simulink model "test_convert"  (Simulink 6.2)
settings: Solver=ode45  StartTime=0.0  StopTime=10.0  RelTol=1e-3
libraries: xbsIndex_r3 x9
settings Model: LastModifiedBy=mdexter
settings DebuggingCC: SolverPrmCheckMsg=warning

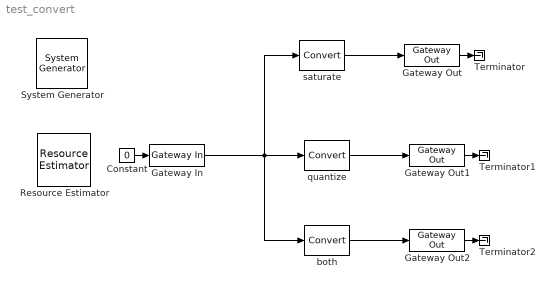
== system test_convert ==
  " System Generator" : xbsIndex_r3/ System Generator  Tag=genX  xilinxfamily=Virtex2  part=xc2v1000  speed=-4  package=bg575  synthesis_tool=XST  directory=./test_convert.netlist  testbench=off  simulink_period=1  sysclk_period=100  incr_netlist=off  trim_vbits=Everywhere in SubSystem  dbl_ovrd=According to Block Masks  core_generation=According to Block Masks  run_coregen=off  deprecated_control=off  eval_field=0
      settings: AttributesFormatString=System\nGenerator
  Constant : Constant  Value=0
  Gateway In : xbsIndex_r3/Gateway In  arith_type="Signed  (2's comp)"  n_bits=18  bin_pt=9  quantization=Truncate  overflow=Wrap  period=1  timing_constraint=None  locs_specified=off  LOCs={}  needs_fixed_name=off  dbl_ovrd=off  show_param=off
      settings: xl_area=[0 0 0 0 18 0 0]
  Gateway Out : xbsIndex_r3/Gateway Out  output_type=Double  nbits=8  bin_pt=6  arith_type=Boolean  quantization=Truncate  overflow=Wrap  hdl_port=on  timing_constraint=None  locs_specified=off  LOCs={}  needs_fixed_name=off  show_param=off
      settings: xl_area=[0 0 0 0 10 0 0]
  Gateway Out1 : xbsIndex_r3/Gateway Out  output_type=Double  nbits=8  bin_pt=6  arith_type=Boolean  quantization=Truncate  overflow=Wrap  hdl_port=on  timing_constraint=None  locs_specified=off  LOCs={}  needs_fixed_name=off  show_param=off
      settings: xl_area=[0 0 0 0 9 0 0]
  Gateway Out2 : xbsIndex_r3/Gateway Out  output_type=Double  nbits=8  bin_pt=6  arith_type=Boolean  quantization=Truncate  overflow=Wrap  hdl_port=on  timing_constraint=None  locs_specified=off  LOCs={}  needs_fixed_name=off  show_param=off
      settings: xl_area=[0 0 0 0 4 0 0]
  Resource Estimator : xbsIndex_r3/Resource Estimator  Tag=resEstTag  xl_estimator_area=[39 23 0 71 41 0 0]  xl_use_estimator_area=off  simulink_period=1  mrp_directory=./bitsel_core
      settings: AttributesFormatString=Resource\nEstimator
  Terminator : Terminator
  Terminator1 : Terminator
  Terminator2 : Terminator
  both : xbsIndex_r3/Convert  arith_type="Signed  (2's comp)"  n_bits=4  bin_pt=0  quantization="Round  (unbiased: Even Values)"  overflow=Saturate  latency=3  explicit_period=off  period=1  dbl_ovrd=off  show_param=on  inserted_by_tool=off  pipeline=on
      settings: AttributesFormatString=%<n_bits>_%<bin_pt> out\n%<xl_area>  xl_area=[13 4 0 26 0 0 0]
  quantize : xbsIndex_r3/Convert  arith_type="Signed  (2's comp)"  n_bits=9  bin_pt=0  quantization="Round  (unbiased: Even Values)"  overflow=Wrap  latency=3  explicit_period=off  period=1  dbl_ovrd=off  show_param=on  inserted_by_tool=off  pipeline=on
      settings: AttributesFormatString=%<n_bits>_%<bin_pt> out\n%<xl_area>  xl_area=[14 9 0 22 0 0 0]
  saturate : xbsIndex_r3/Convert  arith_type="Signed  (2's comp)"  n_bits=10  bin_pt=9  quantization=Truncate  overflow=Saturate  latency=3  explicit_period=off  period=1  dbl_ovrd=off  show_param=on  inserted_by_tool=off  pipeline=on
      settings: AttributesFormatString=%<n_bits>_%<bin_pt> out\n%<xl_area>  xl_area=[12 10 0 23 0 0 0]
  wires:
  Gateway In/1 -> saturate/1, quantize/1, both/1
  saturate/1 -> Gateway Out/1
  Constant/1 -> Gateway In/1
  Gateway Out/1 -> Terminator/1
  quantize/1 -> Gateway Out1/1
  Gateway Out1/1 -> Terminator1/1
  both/1 -> Gateway Out2/1
  Gateway Out2/1 -> Terminator2/1
